simulink model "tankProblemSimu"  (R2020b)
settings: Solver=VariableStepAuto  StartTime=0.0  StopTime=10.0  RelTol=1e-3
values from neighbouring files (symbols this model uses):
  c = 16    [TankFillingScript.m]
undefined symbols (not defined in the file or in its folder): aIn, Q
settings Model: Creator=mreiff  LastModifiedBy=mreiff

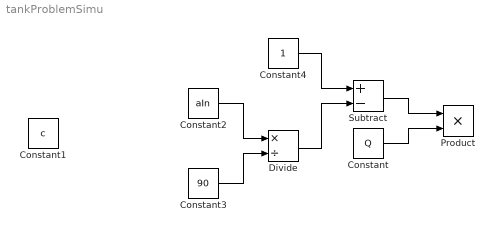
== system tankProblemSimu ==
  Constant : Constant  Value=Q
  Constant1 : Constant  Value=c
  Constant2 : Constant  Value=aIn
  Constant3 : Constant  Value=90
  Constant4 : Constant
  Divide : Product  Inputs=*/
  Product : Product
  Subtract : Sum  Inputs=+-
  wires:
  Constant2/1 -> Divide/1
  Constant3/1 -> Divide/2
  Constant4/1 -> Subtract/1
  Divide/1 -> Subtract/2
  Subtract/1 -> Product/1
  Constant/1 -> Product/2
